simulink model "MEM_model_updated"  (R2020a)
settings: Solver=ode45  StartTime=0.0  StopTime=.5  MaxStep=1e-6  RelTol=1e-3  EnableMultiTasking=on
libraries: simulink x1
settings Model: SimulationMode=accelerator  Creator=OXAALJ  LastModifiedBy=galarm2
settings SolverCC: MaxOrder=2  MaxConsecutiveZCs=10  MaxConsecutiveMinStep=10  ZeroCrossControl=DisableAll
settings DataIOCC: LimitDataPoints=on  SaveFormat=Array  DSMLogging=off  ReturnWorkspaceOutputs=off
settings OptimizationCC: EfficientMapNaN2IntZero=off  LifeSpan=inf
settings DebuggingCC: UnderspecifiedInitializationDetection=Classic  MergeDetectMultiDrivingBlocksExec=none  SolverPrmCheckMsg=warning  MultiTaskDSMMsg=warning  MultiTaskCondExecSysMsg=none  StateNameClashWarn=warning  SFUnexpectedBacktrackingDiag=warning  SFNoUnconditionalDefaultTransitionDiag=warning  SFExecutionAtInitializationDiag=none  ArithmeticOperatorsInVariantConditions=warning
settings HardwareCC: ProdBitPerPointer=32  ProdBitPerSizeT=32  ProdBitPerPtrDiffT=32  ProdLargestAtomicFloat=None  ProdIntDivRoundTo=Undefined  ProdEndianess=Unspecified  ProdWordSize=32  ProdHWDeviceType=32-bit Generic  TargetBitPerPointer=64  TargetBitPerSizeT=64  TargetBitPerPtrDiffT=64  TargetLongLongMode=on  TargetIntDivRoundTo=Zero  TargetEndianess=LittleEndian  TargetWordSize=64  TargetHWDeviceType=MATLAB Host  ProdEqTarget=off
settings ModelReferenceCC: PropagateSignalLabelsOutOfModel=off
settings SFSimCC: SimUseLocalCustomCode=off  CustomCodeUndefinedFunction=UseInterfaceOnly
settings CodeAppCC: MaxIdLength=128
settings GRTTargetCC: TargetLangStandard=C89/C90 (ANSI)  CombineOutputUpdateFcns=off  GRTInterface=on
settings ConfigComp: CovMetricSettings=dw  CovHtmlReporting=on  CovSaveCumulativeToWorkspaceVar=on  CovSaveSingleToWorkspaceVar=on  CovExternalEMLEnable=off  CovSFcnEnable=off

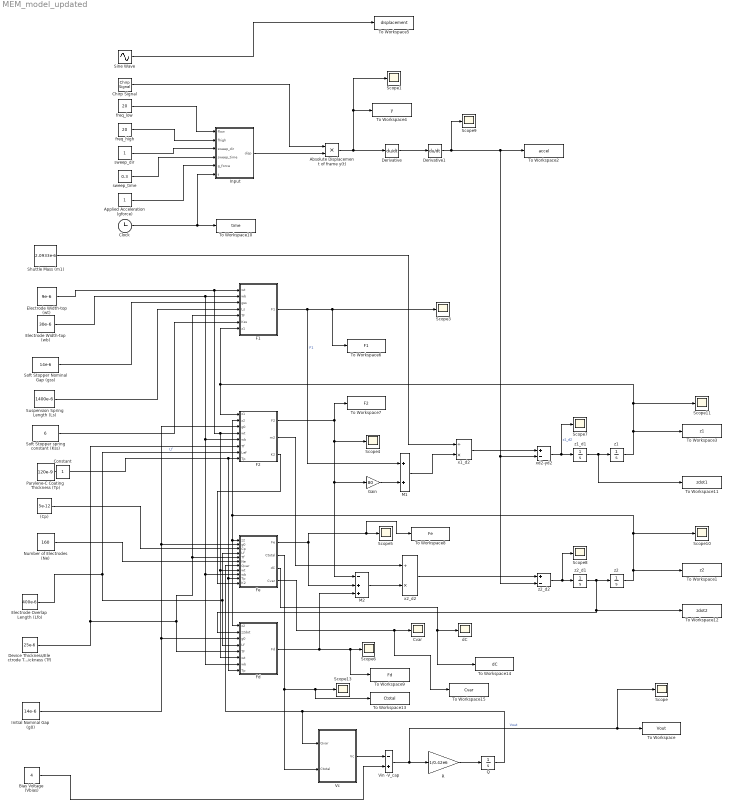
== system MEM_model_updated ==
  " M2" : Sum  Inputs=-++  RndMeth=Nearest
  (Cp) : Constant  Value=5e-12  VectorParams1D=off
  Absolute Displacement of frame y(t) : Product
  Applied Acceleration (gforce) : Constant
  Bias Voltage (Vbias) : Constant  Value=4
  Chirp Signal : simulink/Sources/Chirp Signal  f1=20  T=0.3  f2=20
  Clock : Clock
  Cvar : Scope
  Derivative : Derivative
  Derivative1 : Derivative
  Device Thickness/Electrode Thickness (Tf) : Constant  Value=25e-6
  Electrode Overlap Length (Lfo) : Constant  Value=400e-6
  Electrode Width-top (wb) : Constant  Value=30e-6
  Electrode Width-top (wt) : Constant  Value=9e-6
  F1 : MATLAB Function  TreatAsAtomicUnit=on
  F2 : MATLAB Function  TreatAsAtomicUnit=on
  Fd : MATLAB Function  TreatAsAtomicUnit=on
  Fe : MATLAB Function  TreatAsAtomicUnit=on
  Gain : Gain  Gain=80
  Initial Nominal Gap (g0) : Constant  Value=14e-6
  Input : MATLAB Function  TreatAsAtomicUnit=on
  M1 : Sum  RndMeth=Nearest
  Number of Electrodes (Ne) : Constant  Value=160
  Parylene-C Coating Thickness (Tp) : Constant  Value=120e-9
  Q : Integrator
  R : Gain  Gain=1/0.42e6
  Scope{,1,3..11,13} (12 alike) : Scope
  Shuttle Mass (m1) : Constant  Value=2.0933e-6
  Sine Wave : Sin  Amplitude=9.81  Frequency=6.28*20  SampleTime=0
  Soft Stopper Nominal Gap (gss) : Constant  Value=14e-6
  Soft Stopper spring constant (Kss) : Constant  Value=6
  Suspension Spring Length (Ls) : Constant  Value=1400e-6
  To Workspace : ToWorkspace  VariableName=Vout  SampleTime=-1
      settings: Save2DSignal=2-D array (concatenate along first dimension)
  To Workspace1 : ToWorkspace  VariableName=z2  SampleTime=-1
      settings: Save2DSignal=2-D array (concatenate along first dimension)
  To Workspace10 : ToWorkspace  VariableName=time  SampleTime=-1
      settings: Save2DSignal=2-D array (concatenate along first dimension)
  To Workspace11 : ToWorkspace  VariableName=zdot1  SampleTime=-1
      settings: Save2DSignal=2-D array (concatenate along first dimension)
  To Workspace12 : ToWorkspace  VariableName=zdot2  SampleTime=-1
      settings: Save2DSignal=2-D array (concatenate along first dimension)
  To Workspace13 : ToWorkspace  VariableName=Ctotal  SampleTime=-1
      settings: Save2DSignal=2-D array (concatenate along first dimension)
  To Workspace14 : ToWorkspace  VariableName=dC  SampleTime=-1
      settings: Save2DSignal=2-D array (concatenate along first dimension)
  To Workspace15 : ToWorkspace  VariableName=Cvar  SampleTime=-1
      settings: Save2DSignal=2-D array (concatenate along first dimension)
  To Workspace2 : ToWorkspace  VariableName=accel  SampleTime=-1
      settings: Save2DSignal=2-D array (concatenate along first dimension)
  To Workspace3 : ToWorkspace  VariableName=z1  SampleTime=-1
      settings: Save2DSignal=2-D array (concatenate along first dimension)
  To Workspace4 : ToWorkspace  VariableName=y  SampleTime=-1
      settings: Save2DSignal=2-D array (concatenate along first dimension)
  To Workspace5 : ToWorkspace  VariableName=displacement  SampleTime=-1
      settings: Save2DSignal=2-D array (concatenate along first dimension)
  To Workspace6 : ToWorkspace  VariableName=F1  SampleTime=-1
      settings: Save2DSignal=2-D array (concatenate along first dimension)
  To Workspace7 : ToWorkspace  VariableName=F2  SampleTime=-1
      settings: Save2DSignal=2-D array (concatenate along first dimension)
  To Workspace8 : ToWorkspace  VariableName=Fe  SampleTime=-1
      settings: Save2DSignal=2-D array (concatenate along first dimension)
  To Workspace9 : ToWorkspace  VariableName=Fd  SampleTime=-1
      settings: Save2DSignal=2-D array (concatenate along first dimension)
  Vc : MATLAB Function  TreatAsAtomicUnit=on
  Vin -V_cap : Sum  Inputs=-+  RndMeth=Nearest
  dC : Scope
  freq_high : Constant  Value=20
  freq_low : Constant  Value=20
  sweep_dir : Constant
  sweep_time : Constant  Value=0.3
  x1_d2 : Product  Inputs=/*
  x2_d2 : Product  Inputs=/*
  xd2-yd2 : Sum  Inputs=+-  RndMeth=Nearest
  z1 : Integrator
  z1_d1 : Integrator
  z2 : Integrator
  z2_d1 : Integrator
  z2_d2 : Sum  Inputs=+-  RndMeth=Nearest
  Constant : Constant  IOType=siggen
  wires:
  F1/1(F1) -> M1/1, To Workspace6/1, Scope3/1  "F1"
  Shuttle Mass (m1)/1 -> x1_d2/1
  Initial Nominal Gap (g0)/1 -> F2/3(g0), Fe/2(g0), Fd/3(g0)
  Bias Voltage (Vbias)/1 -> Vin -V_cap/2
  Vin -V_cap/1 -> Scope/1, To Workspace/1, R/1  "Vout"
  R/1 -> Q/1
  Q/1 -> Fe/7(Qvar), Vc/1(Qvar)
  Electrode Overlap Length (Lfo)/1 -> F2/7(Lef), Fd/4(Lf), Fe/4(Lf)  "Lf"
  (Cp)/1 -> Fe/3(Cp)
  Suspension Spring Length (Ls)/1 -> F1/4(Ls)
  Device Thickness/Electrode Thickness (Tf)/1 -> F2/6(Tf), Fd/5(Tf), F1/5(Tf), Fe/5(Tf)
  Soft Stopper spring constant (Kss)/1 -> F1/6(Kss)
  M1/1 -> x1_d2/2
  x1_d2/1 -> xd2-yd2/1
  xd2-yd2/1 -> Scope7/1, z1_d1/1  "z1_d2"
  z1_d1/1 -> To Workspace11/1, z1/1
  x2_d2/1 -> z2_d2/1
  z2_d1/1 -> To Workspace12/1, Fd/2(z2dot), z2/1
  z2/1 -> Scope10/1, Fd/1(z2), Fe/1(z2), F2/2(z2), To Workspace1/1
  " M2"/1 -> x2_d2/2
  Soft Stopper Nominal Gap (gss)/1 -> F1/3(gss)
  Input/1(disp) -> Absolute Displacement of frame y(t)/2
  freq_high/1 -> Input/2(fhigh)
  Applied Acceleration (gforce)/1 -> Input/5(g_force)
  Clock/1 -> To Workspace10/1, Input/6(t)
  F2/1(F2) -> To Workspace7/1, Scope4/1, Gain/1, " M2"/1
  F2/2(m2) -> x2_d2/1
  Parylene-C Coating Thickness (Tp)/1 -> Fd/8(Tp), Fe/10(Tp), F2/8(Tp)
  Fe/1(Fe) -> To Workspace8/1, Scope5/1, " M2"/2
  Fe/2(Ctotal) -> Vc/2(Ctotal), To Workspace13/1, Scope13/1
  Fd/1(Fd) -> " M2"/3, To Workspace9/1, Scope6/1
  Vc/1(Vc) -> Vin -V_cap/1
  Electrode Width-top (wt)/1 -> Fd/6(wt), Fe/8(wt), F2/4(wt), F1/1(wt)
  Electrode Width-top (wb)/1 -> Fd/7(wb), Fe/9(wb), F2/5(wb), F1/2(wb)
  Absolute Displacement of frame y(t)/1 -> Scope1/1, To Workspace4/1, Derivative/1
  Derivative/1 -> Derivative1/1
  freq_low/1 -> Input/1(flow)
  sweep_time/1 -> Input/4(sweep_time)
  sweep_dir/1 -> Input/3(sweep_dir)
  z2_d2/1 -> Scope8/1, z2_d1/1
  Derivative1/1 -> To Workspace2/1, z2_d2/2, xd2-yd2/2, Scope9/1
  Gain/1 -> M1/2
  z1/1 -> Scope11/1, F2/1(z1), F1/7(z1), To Workspace3/1
  Number of Electrodes (Ne)/1 -> Fe/6(Ne)
  Fe/3(dC) -> To Workspace14/1, dC/1
  Fe/4(Cvar) -> To Workspace15/1, Cvar/1
  F2/3(K2) -> Fe/11(K2)
  Chirp Signal/1 -> Absolute Displacement of frame y(t)/1
  Sine Wave/1 -> To Workspace5/1

== matlab function MEM_model_updated/Fd ==
  data: z2 input; z2dot input; g0 input; Fd output; Lf input; Tf input; wt input; wb input; Tp input
function Fd = fcn(z2,z2dot,g0,Lf,Tf,wt,wb,Tp)
% This function calculates the force F2
% Device Parameters
gp = g0 - 2*Tp; % minimum air gap 
eta = 1.849e-5; % Dynamic viscosity of air (kg/m*s)
a = (wb-wt)/Lf;
% Lf = Lf + 50e-6;

% Scaling term for Damping force
set = 0;
if abs(z2) >= gp
    set = set + 1;
end

if set < 1
    scale = 0.015; % Scaling term for Damping force
else
    scale = 0.01965; 
end

% Fd_l
ul  =  gp + z2; % Left-hand side ho
ll  =  ul + a*Lf; % Left-hand side hl
A1_l  =  -ul*Lf/(ul + 2*a)* z2dot; % The c1 parameter, left
A2_l  =  12*eta*a^-2/(2*ul + a*Lf) * z2dot; % The c1 parameter, left
Fd_l   =  Tf*(Lf*A2_l - 6*eta*Lf/a/ul/ll*A1_l + 6*eta*Lf*a^-4/ll*z2dot + 12*eta*a^-3 * z2dot * (log(abs(ul./ll))) );

% Fd_r
ur  =  gp - z2;  
lr  =  ur + a*Lf;
A1_r  =  -ur*Lf/(ur + 2*a)* z2dot; % The c1 parameter, right
A2_r  =  12*eta*a^-2/(2*ur + a*Lf) * z2dot; % The c1 parameter, right
Fd_r   =  Tf*(Lf*A2_r - 6*eta*Lf/a/ur/lr*A1_r + 6*eta*Lf*a^-4/lr*z2dot - 12*eta*a^-3 * z2dot * (log(abs(ur./lr))) );

% Fd
Fd  =  -scale*(Fd_l + Fd_r);
end

== matlab function MEM_model_updated/Vc ==
  data: Qvar input; Vc output; Ctotal input
function Vc = fcn(Qvar,Ctotal)
% This function calculates the Vc value
Vc = Qvar/Ctotal;
end

== matlab function MEM_model_updated/Fe ==
  data: z2 input; g0 input; Cp input; Fe output; Lf input; Tf input; Ne input; Qvar input; wt input; wb input; Tp input; Ctotal output; dC output; Cvar output; K2 input
function [Fe,Ctotal,dC,Cvar] = fcn(z2,g0,Cp,Lf,Tf,Ne,Qvar,wt,wb,Tp,K2)
% This function calculates the force F2
% Device Parameters
gp = g0 - 2*Tp; % minimum air gap 
ws = mean([wt,wb]); % Avg. Electrode width
I = (1/12)*Tf*(ws^3); % Moment of Inertia average width
E = 180e9; % The Young's modulous 
e = 8.85e-12; % Permittivity of free space
ep = 3.2; % Relative Permittivity of Parylene-C
% ws = 0.5*(wt + wb); % Avg. electrode width
a = (wb-wt)/Lf;
scale = 1;
% Lf = Lf + 50e-6;
Cvar = 0;

if abs(z2) < gp % The electrodes are not in contact
    % Cvar_r
    Crl = (ep.*e.*Lf.*Tf)/Tp;
    Cair_r = ((e.*Tf)/(2.*a)).*(log((g0 - z2 + 2.*a.*Lf)./(g0 - z2)));
    Cvar_r = 1/((1/Crl)+(1/Cair_r)+(1/Crl));
    % Cvar_l
    Cair_l = ((e.*Tf)./(2.*a)).*(log((g0 + z2 + 2.*a.*Lf)./(g0 + z2)));
    Cvar_l = 1./((1/Crl)+(1/Cair_l)+(1/Crl));
    % Cvar
    Cvar = (Cvar_r + Cvar_l).*(Ne/2);
elseif abs(z2) >= gp % The electrodes are in contact
    % Colliding Electrode
    Crl = (ep.*e.*Lf.*Tf)/Tp;
    d = (wb-wt)-(((K2*(abs(z2)-g0))*(Lf^3))/(3*E*I));
    % Cair_c = ((e*Tf*(Lf^2))/(2*d))*(log(abs(d-2*Tp))-log(abs((2*Tp))));
    % Cair_c = ((e*Tf*Lf)/(2*d))*(log((2*Tp + 2*d)/(2*Tp)));
    Cair_c = ((e*Tf*Lf)/(d))*(log((2*Tp + 2*d)/(2*Tp)));
    Cvar_c = 1./((1/Crl)+(1/Cair_c)+(1/Crl));
    % Non-colliding Electrode
    Cair_nc = ((e.*Tf)./(2.*a)).*(log((g0 + abs(z2) + 2.*a.*Lf)./(g0 + abs(z2))));
    Cvar_nc = 1./((1/Crl)+(1/Cair_nc)+(1/Crl));
    % Cvar
    Cvar = (Cvar_nc + Cvar_c).*(Ne/2);     
end

% Ctotal
Ctotal = Cvar + Cp;

% dC is divided by four here because nf is total electrodes, not number of electrode pairs
dC = ((e*Ne*Tf)./(4.*a))*( ((2*z2)/(gp^2 - z2^2)) - ((2*z2)/((gp + 2*Lf*a)^2 - z2^2) ));
% dC = ((e*Ne*Lf)./(4.*a))*( ((2*z2)/(g0^2 - z2^2)) - ((2*z2)/((g0 + 2*Tf*a)^2 - z2^2) ));

% Fe
NFe = -1*((Qvar^2)/(2*Ctotal^2))*dC;
Fe = NFe./(Ne/2)*scale;
end

== matlab function MEM_model_updated/Input ==
  data: flow input; fhigh input; sweep_dir input; sweep_time input; g_force input; disp output; t input
function disp  = fcn(flow,fhigh,sweep_dir,sweep_time,g_force,t)
ramp = 200e-3;

if sweep_dir > 0
    %upsweep
    if t < ramp
        freq = (t/sweep_time)*(fhigh-flow) + flow;
        disp = (t/ramp)* (g_force/(4.0243*freq^2)); %const = (2*pi())^2/9.81
        % vel = (t/ramp)*(g_force*9.81)/(2*pi*freq);
    else
        freq = (t/sweep_time)*(fhigh-flow) + flow;
        disp = g_force/(4.0243*freq^2);   %const = (2*pi())^2/9.81
        % vel = (g_force*9.81)/(2*pi*freq);
        % disp = g/(4.0243*((fhigh-flow)/2)^2); 
        % freq = (0.5) * (fhigh+flow);
        % disp = g/(4.0243*freq^2);  %const = (2*pi())^2/9.81
    end
else
    %downsweep
    if t < ramp
        freq = fhigh - (t/sweep_time)*(fhigh-flow);
        disp = (t/ramp)* (g_force/(4.0243*freq^2)); %const = (2*pi())^2/9.81
        % vel = (t/ramp)*(g_force*9.81)/(2*pi*freq);
    else
        freq = fhigh - (t/sweep_time)*(fhigh-flow);
        disp = g_force/(4.0243*freq^2);  %const = (2*pi())^2/9.81
        % vel = (g_force*9.81)/(2*pi*freq);
        % disp = g/(4.0243*((fhigh-flow)/2)^2); 
        % freq = (0.5) * (fhigh+flow);
        % disp = g/(4.0243*freq^2);  %const = (2*pi())^2/9.81
    end
end
end

== matlab function MEM_model_updated/F2 ==
  data: z1 input; z2 input; F2 output; g0 input; m2 output; wt input; wb input; Tf input; Lef input; Tp input; K2 output
function [F2,m2,K2] = fcn(z1,z2,g0,wt,wb,Tf,Lef,Tp)
% This function calculates the force F2
% Device Parameters
gp = g0 - 2*Tp; % minimum air gap
E = 180e9; % The Young's modulous 
rho = 2333; % density (kg/m3)
ws = mean([wt,wb]); % Avg. Electrode width
Lf = Lef + 50e-6; % Account for non-overlap
I = (1/12)*Tf*(ws^3); % Moment of Inertia average width
% h = (wb-wt)*(Lef/Lf); % height function
% I = (1/12)*Tf*(h^3); % Moment of Inertia height function

% NF2 and Nm2
if abs(z2) < gp
    m2 = (33/140)*rho*Tf*Lf*ws; % Mass of single electrode
    K2 = (1/4)*E/Lf^3*I; % Spring constant of electrode
    % K2 = 135801;
    F2 = -K2*(z1-z2);
  
else    
    m2 = 2*(33/140)*rho*Tf*Lf*ws; % Mass of combined electrode
    K2 = (1/4)*E/Lf^3*I; % Spring constant of electrode
    % K2 = 135801;
    % F2 = -K2*(z1-z2);
    F2 = -K2*(z1-z2) + K2*(abs(z2)-gp)*sign(z2);
end
end

== matlab function MEM_model_updated/F1 ==
  data: wt input; wb input; gss input; Ls input; Tf input; Kss input; z1 input; F1 output
function F1 = fcn(wt,wb,gss,Ls,Tf,Kss,z1)
% This function calculates the force F1
% Device Parameters
E = 180e9; % The Young's modulous

% Fsp
% omega0 = Fres*2*pi; % The measured resonant angular frequency                       
% k1 = (omega0)^2*m1; % Linear spring constant k1 (N/m)
% ws_effective = (((Ls^3)*k1)/(2*E*Tf))^(1/3); % Effective spring beam width (m)
% k3_single = (18/25)*(k1/2)*(1/(ws_effective^2)); % Cubic spring constant of a single spring k3 (N/m)
% k3 = k3_single/8; % k3 of all the connected suspension springs

ws = 14.7e-6;
% ws = mean([wt,wb]); % Avg. electrode width
k1 = (4/6)*((E*Tf*(ws^3))/(Ls^3)); % Spring constant from supporting beams
k3 = (18/25)*((E*Tf*ws)/(Ls^3)); % cubic spring constant

Fsp = 0.01*(-k1.*z1 - k3.*(z1^3)); % suspension beam force
% Fsp = (-k1.*z1); % suspension beam force

% Fss
if abs(z1) < gss
    Fss = 0; % stopper not engaged
else
    Fss = Kss*(abs(z1)-gss)*sign(z1); % stopper is engaged
end

F1 = Fss + Fsp;
end
